simulink model "xue_flatness"  (R2017b)
settings: Solver=VariableStepAuto  StartTime=0.0  StopTime=58  RelTol=1e-9
libraries: simulink x1
(part 2 of 3)

== matlab function xue_flatness/References ==
  data: t input; references output size=18
function references = fcn(t)
%% specify your references here
g=9.81;
if t>=0 && t<2
tanalpha=-1;
if t>=0 && t<1
   [ax_d, az_d, ax_d_dot, az_d_dot, ax_d_dot_dot, az_d_dot_dot]=nest(t);
    ax_d=2/3*ax_d;                   az_d=2/3*az_d;
    ax_d_dot=2/3*ax_d_dot;           az_d_dot=2/3*az_d_dot;
    ax_d_dot_dot=2/3*ax_d_dot_dot;   az_d_dot_dot=2/3*az_d_dot_dot;
else % t>=1 && t<2
   [ax_d, az_d, ax_d_dot, az_d_dot, ax_d_dot_dot, az_d_dot_dot]=nest(t-1);
  ax_d=-2/3*ax_d;                 az_d=-2/3*az_d; % invert the direction for the sake of making end velocity zero
  ax_d_dot=-2/3*ax_d_dot;         az_d_dot=-2/3*az_d_dot;
  ax_d_dot_dot=-2/3*ax_d_dot_dot; az_d_dot_dot=-2/3*az_d_dot_dot;   
end  
 r_desired=[0 0 0]'    ;              % reference's positions is not solved here
 r_desired_dot=[0 0 0]'    ;          % reference's velocities is not solved here
 r_desired_dot_dot=[ax_d 0 az_d]'   ;       % reference's accelerations
 r_desired_dot_dot_dot=[ax_d_dot 0 az_d_dot]';      % jerk
 r_desired_dot_dot_dot_dot=[ax_d_dot_dot 0 az_d_dot_dot]' ; % snap
 psi_desired=0 ;                      % reference's yaw angle
 psi_desired_dot=0 ;                  % reference's change rate of yaw angle       
 psi_desired_dot_dot=0;
 
elseif t>=2 && t<4
r_desired=[0 0 0]'    ;              % reference's positions is not solved here
r_desired_dot=[0 0 0]'    ;          % reference's velocities is not solved here
r_desired_dot_dot=[0 0 0]'   ;       % reference's accelerations
r_desired_dot_dot_dot=[0 0 0]';      % jerk
r_desired_dot_dot_dot_dot=[0 0 0]' ; % snap
if t>=2 && t<3
psi_desired=pi/4*(t-2)^2 ;                      % reference's yaw angle
psi_desired_dot=pi/2*(t-2);                  % reference's change rate of yaw angle       
psi_desired_dot_dot=pi/2; 
else % t>=3 && t<4
psi_desired=-pi/4*(t-4)^2+pi/2 ;                      % reference's yaw angle
psi_desired_dot=-pi/2*(t-4);                  % reference's change rate of yaw angle       
psi_desired_dot_dot=-pi/2; 
end

elseif t>=4 && t<6
tanalpha=1;
if t>=4 && t<5
   [ax_d, az_d, ax_d_dot, az_d_dot, ax_d_dot_dot, az_d_dot_dot]=nest(t-4);
    ax_d=2/3*ax_d;                   az_d=2/3*az_d;
    ax_d_dot=2/3*ax_d_dot;           az_d_dot=2/3*az_d_dot;
    ax_d_dot_dot=2/3*ax_d_dot_dot;   az_d_dot_dot=2/3*az_d_dot_dot;
else % t>=5 && t<6
   [ax_d, az_d, ax_d_dot, az_d_dot, ax_d_dot_dot, az_d_dot_dot]=nest(t-5);
  ax_d=-2/3*ax_d;                 az_d=-2/3*az_d; % invert the direction for the sake of making end velocity zero
  ax_d_dot=-2/3*ax_d_dot;         az_d_dot=-2/3*az_d_dot;
  ax_d_dot_dot=-2/3*ax_d_dot_dot; az_d_dot_dot=-2/3*az_d_dot_dot;   
end  
 r_desired=[0 0 0]'    ;              % reference's positions is not solved here
 r_desired_dot=[0 0 0]'    ;          % reference's velocities is not solved here
 r_desired_dot_dot=[ax_d 0 az_d]'   ;       % reference's accelerations
 r_desired_dot_dot_dot=[ax_d_dot 0 az_d_dot]';      % jerk
 r_desired_dot_dot_dot_dot=[ax_d_dot_dot 0 az_d_dot_dot]' ; % snap
 psi_desired=pi/2 ;                      % reference's yaw angle
 psi_desired_dot=0 ;                  % reference's change rate of yaw angle       
 psi_desired_dot_dot=0;

elseif t>=6 && t<8
r_desired=[0 0 0]'    ;              % reference's positions is not solved here
r_desired_dot=[0 0 0]'    ;          % reference's velocities is not solved here
r_desired_dot_dot=[0 0 0]'   ;       % reference's accelerations
r_desired_dot_dot_dot=[0 0 0]';      % jerk
r_desired_dot_dot_dot_dot=[0 0 0]' ; % snap
if t>=6 && t<7
psi_desired=pi/2-pi/4*(t-6)^2 ;                      % reference's yaw angle
psi_desired_dot=-pi/2*(t-6);                  % reference's change rate of yaw angle       
psi_desired_dot_dot=-pi/2; 
else % t>=7 & t<8
psi_desired=pi/4*(t-8)^2 ;                      % reference's yaw angle
psi_desired_dot=pi/2*(t-8);                  % reference's change rate of yaw angle       
psi_desired_dot_dot=pi/2; 
end

elseif t>=8 && t<10
tanalpha=-1;
if t>=8 && t<9
   [ax_d, az_d, ax_d_dot, az_d_dot, ax_d_dot_dot, az_d_dot_dot]=nest(t-8);
    ax_d=2/3*ax_d;                   az_d=2/3*az_d;
    ax_d_dot=2/3*ax_d_dot;           az_d_dot=2/3*az_d_dot;
    ax_d_dot_dot=2/3*ax_d_dot_dot;   az_d_dot_dot=2/3*az_d_dot_dot;
else % t>=9 && t<10
   [ax_d, az_d, ax_d_dot, az_d_dot, ax_d_dot_dot, az_d_dot_dot]=nest(t-9);
  ax_d=-2/3*ax_d;                 az_d=-2/3*az_d; % invert the direction for the sake of making end velocity zero
  ax_d_dot=-2/3*ax_d_dot;         az_d_dot=-2/3*az_d_dot;
  ax_d_dot_dot=-2/3*ax_d_dot_dot; az_d_dot_dot=-2/3*az_d_dot_dot;   
end  
 r_desired=[0 0 0]'    ;              % reference's positions is not solved here
 r_desired_dot=[0 0 0]'    ;          % reference's velocities is not solved here
 r_desired_dot_dot=[ax_d 0 az_d]'   ;       % reference's accelerations
 r_desired_dot_dot_dot=[ax_d_dot 0 az_d_dot]';      % jerk
 r_desired_dot_dot_dot_dot=[ax_d_dot_dot 0 az_d_dot_dot]' ; % snap
 psi_desired=0 ;                      % reference's yaw angle
 psi_desired_dot=0 ;                  % reference's change rate of yaw angle       
 psi_desired_dot_dot=0;
 
elseif t>=10 && t<12
r_desired=[0 0 0]'    ;              % reference's positions is not solved here
r_desired_dot=[0 0 0]'    ;          % reference's velocities is not solved here
r_desired_dot_dot=[0 0 0]'   ;       % reference's accelerations
r_desired_dot_dot_dot=[0 0 0]';      % jerk
r_desired_dot_dot_dot_dot=[0 0 0]' ; % snap
if t>=10 && t<11
psi_desired=pi/4*(t-10)^2 ;                      % reference's yaw angle
psi_desired_dot=pi/2*(t-10);                  % reference's change rate of yaw angle       
psi_desired_dot_dot=pi/2; 
else % t>=11 && t<12
psi_desired=-pi/4*(t-12)^2+pi/2 ;                      % reference's yaw angle
psi_desired_dot=-pi/2*(t-12);                  % reference's change rate of yaw angle       
psi_desired_dot_dot=-pi/2; 
end

elseif t>=12 && t<14
tanalpha=0.5;
if t>=12 && t<13
   [ax_d, az_d, ax_d_dot, az_d_dot, ax_d_dot_dot, az_d_dot_dot]=nest(t-12);
    ax_d=406/329*ax_d;                   az_d=406/329*az_d;
    ax_d_dot=406/329*ax_d_dot;           az_d_dot=406/329*az_d_dot;
    ax_d_dot_dot=406/329*ax_d_dot_dot;   az_d_dot_dot=406/329*az_d_dot_dot;
else % t>=13 && t<14
   [ax_d, az_d, ax_d_dot, az_d_dot, ax_d_dot_dot, az_d_dot_dot]=nest(t-13);
  ax_d=-406/329*ax_d;                 az_d=-406/329*az_d; % invert the direction for the sake of making end velocity zero
  ax_d_dot=-406/329*ax_d_dot;         az_d_dot=-406/329*az_d_dot;
  ax_d_dot_dot=-406/329*ax_d_dot_dot; az_d_dot_dot=-406/329*az_d_dot_dot;   
end  
 r_desired=[0 0 0]'    ;              % reference's positions is not solved here
 r_desired_dot=[0 0 0]'    ;          % reference's velocities is not solved here
 r_desired_dot_dot=[ax_d 0 az_d]'   ;       % reference's accelerations
 r_desired_dot_dot_dot=[ax_d_dot 0 az_d_dot]';      % jerk
 r_desired_dot_dot_dot_dot=[ax_d_dot_dot 0 az_d_dot_dot]' ; % snap
 psi_desired=pi/2 ;                      % reference's yaw angle
 psi_desired_dot=0 ;                  % reference's change rate of yaw angle       
 psi_desired_dot_dot=0;
 
elseif t>=14 && t<16
r_desired=[0 0 0]'    ;              % reference's positions is not solved here
r_desired_dot=[0 0 0]'    ;          % reference's velocities is not solved here
r_desired_dot_dot=[0 0 0]'   ;       % reference's accelerations
r_desired_dot_dot_dot=[0 0 0]';      % jerk
r_desired_dot_dot_dot_dot=[0 0 0]' ; % snap
if t>=14 && t<15
psi_desired=pi/2-pi/4*(t-14)^2 ;                      % reference's yaw angle
psi_desired_dot=-pi/2*(t-14);                  % reference's change rate of yaw angle       
psi_desired_dot_dot=-pi/2; 
else % t>=15 & t<16
psi_desired=pi/4*(t-16)^2 ;                      % reference's yaw angle
psi_desired_dot=pi/2*(t-16);                  % reference's change rate of yaw angle       
psi_desired_dot_dot=pi/2; 
end    

elseif t>=16 && t<18
tanalpha=1;
if t>=16 && t<17
   [ax_d, az_d, ax_d_dot, az_d_dot, ax_d_dot_dot, az_d_dot_dot]=nest(t-16);
    ax_d=-2/3*ax_d;                   az_d=-2/3*az_d;
    ax_d_dot=-2/3*ax_d_dot;           az_d_dot=-2/3*az_d_dot;
    ax_d_dot_dot=-2/3*ax_d_dot_dot;   az_d_dot_dot=-2/3*az_d_dot_dot;
else % t>=17 && t<18
   [ax_d, az_d, ax_d_dot, az_d_dot, ax_d_dot_dot, az_d_dot_dot]=nest(t-17);
  ax_d=2/3*ax_d;                 az_d=2/3*az_d; % invert the direction for the sake of making end velocity zero
  ax_d_dot=2/3*ax_d_dot;         az_d_dot=2/3*az_d_dot;
  ax_d_dot_dot=2/3*ax_d_dot_dot; az_d_dot_dot=2/3*az_d_dot_dot;   
end  
 r_desired=[0 0 0]'    ;              % reference's positions is not solved here
 r_desired_dot=[0 0 0]'    ;          % reference's velocities is not solved here
 r_desired_dot_dot=[ax_d 0 az_d]'   ;       % reference's accelerations
 r_desired_dot_dot_dot=[ax_d_dot 0 az_d_dot]';      % jerk
 r_desired_dot_dot_dot_dot=[ax_d_dot_dot 0 az_d_dot_dot]' ; % snap
 psi_desired=0 ;                      % reference's yaw angle
 psi_desired_dot=0 ;                  % reference's change rate of yaw angle       
 psi_desired_dot_dot=0;   
 
elseif t>=18 && t<20
r_desired=[0 0 0]'    ;              % reference's positions is not solved here
r_desired_dot=[0 0 0]'    ;          % reference's velocities is not solved here
r_desired_dot_dot=[0 0 0]'   ;       % reference's accelerations
r_desired_dot_dot_dot=[0 0 0]';      % jerk
r_desired_dot_dot_dot_dot=[0 0 0]' ; % snap
if t>=18 && t<19
psi_desired=pi/4*(t-18)^2 ;                      % reference's yaw angle
psi_desired_dot=pi/2*(t-18);                  % reference's change rate of yaw angle       
psi_desired_dot_dot=pi/2; 
else % t>=19 && t<20
psi_desired=-pi/4*(t-20)^2+pi/2 ;                      % reference's yaw angle
psi_desired_dot=-pi/2*(t-20);                  % reference's change rate of yaw angle       
psi_desired_dot_dot=-pi/2; 
end

elseif t>=20 && t<22
tanalpha=1/8;
if t>=20 && t<21
   [ax_d, az_d, ax_d_dot, az_d_dot, ax_d_dot_dot, az_d_dot_dot]=nest(t-20);
    ax_d=-8/3*ax_d;                   az_d=-8/3*az_d;
    ax_d_dot=-8/3*ax_d_dot;           az_d_dot=-8/3*az_d_dot;
    ax_d_dot_dot=-8/3*ax_d_dot_dot;   az_d_dot_dot=-8/3*az_d_dot_dot;
else % t>=21 && t<22
   [ax_d, az_d, ax_d_dot, az_d_dot, ax_d_dot_dot, az_d_dot_dot]=nest(t-21);
  ax_d=8/3*ax_d;                 az_d=8/3*az_d; % invert the direction for the sake of making end velocity zero
  ax_d_dot=8/3*ax_d_dot;         az_d_dot=8/3*az_d_dot;
  ax_d_dot_dot=8/3*ax_d_dot_dot; az_d_dot_dot=8/3*az_d_dot_dot;   
end  
 r_desired=[0 0 0]'    ;              % reference's positions is not solved here
 r_desired_dot=[0 0 0]'    ;          % reference's velocities is not solved here
 r_desired_dot_dot=[ax_d 0 az_d]'   ;       % reference's accelerations
 r_desired_dot_dot_dot=[ax_d_dot 0 az_d_dot]';      % jerk
 r_desired_dot_dot_dot_dot=[ax_d_dot_dot 0 az_d_dot_dot]' ; % snap
 psi_desired=pi/2 ;                      % reference's yaw angle
 psi_desired_dot=0 ;                  % reference's change rate of yaw angle       
 psi_desired_dot_dot=0; 
 
elseif t>=22 && t<24
r_desired=[0 0 0]'    ;              % reference's positions is not solved here
r_desired_dot=[0 0 0]'    ;          % reference's velocities is not solved here
r_desired_dot_dot=[0 0 0]'   ;       % reference's accelerations
r_desired_dot_dot_dot=[0 0 0]';      % jerk
r_desired_dot_dot_dot_dot=[0 0 0]' ; % snap
if t>=22 && t<23
psi_desired=pi/2-pi/4*(t-22)^2 ;                      % reference's yaw angle
psi_desired_dot=-pi/2*(t-22);                  % reference's change rate of yaw angle       
psi_desired_dot_dot=-pi/2; 
else % t>=23 & t<24
psi_desired=pi/4*(t-24)^2 ;                      % reference's yaw angle
psi_desired_dot=pi/2*(t-24);                  % reference's change rate of yaw angle       
psi_desired_dot_dot=pi/2; 
end

elseif t>=24 && t<26
if t>=24 && t<25
 r_desired=[0 0 0]'    ;              % reference's positions 
 r_desired_dot=[0 0 0]'    ;          % reference's velocities
 r_desired_dot_dot=[0 0 -1/4]'   ;       % reference's accelerations
 r_desired_dot_dot_dot=[0 0 0]';      % jerk
 r_desired_dot_dot_dot_dot=[0 0 0]' ; % snap
else
 r_desired=[0 0 0]'    ;     % reference's positions 
 r_desired_dot=[0 0 0]'    ;   % reference's velocities 
 r_desired_dot_dot=[0 0 1/4]'   ;       % reference's accelerations
 r_desired_dot_dot_dot=[0 0 0]';      % jerk
 r_desired_dot_dot_dot_dot=[0 0 0]' ; % snap
end
 psi_desired=0 ;                      % reference's yaw angle
 psi_desired_dot=0 ;                  % reference's change rate of yaw angle       
 psi_desired_dot_dot=0;
 
elseif t>=26 && t<28
r_desired=[0 0 0]'    ;              % reference's positions is not solved here
r_desired_dot=[0 0 0]'    ;          % reference's velocities is not solved here
r_desired_dot_dot=[0 0 0]'   ;       % reference's accelerations
r_desired_dot_dot_dot=[0 0 0]';      % jerk
r_desired_dot_dot_dot_dot=[0 0 0]' ; % snap
if t>=26 && t<27
psi_desired=pi/4*(t-26)^2 ;                      % reference's yaw angle
psi_desired_dot=pi/2*(t-26);                  % reference's change rate of yaw angle       
psi_desired_dot_dot=pi/2; 
else % t>=27 && t<28
psi_desired=-pi/4*(t-28)^2+pi/2 ;                      % reference's yaw angle
psi_desired_dot=-pi/2*(t-28);                  % reference's change rate of yaw angle       
psi_desired_dot_dot=-pi/2; 
end

elseif t>=28 && t<30
if t>=28 && t<29
 r_desired=[0 0 0]'    ;              % reference's positions 
 r_desired_dot=[0 0 0]'    ;          % reference's velocities
 r_desired_dot_dot=[0 0 1/4]'   ;       % reference's accelerations
 r_desired_dot_dot_dot=[0 0 0]';      % jerk
 r_desired_dot_dot_dot_dot=[0 0 0]' ; % snap
else
 r_desired=[0 0 0]'    ;     % reference's positions 
 r_desired_dot=[0 0 0]'    ;   % reference's velocities 
 r_desired_dot_dot=[0 0 -1/4]'   ;       % reference's accelerations
 r_desired_dot_dot_dot=[0 0 0]';      % jerk
 r_desired_dot_dot_dot_dot=[0 0 0]' ; % snap
end
 psi_desired=pi/2 ;                      % reference's yaw angle
 psi_desired_dot=0 ;                  % reference's change rate of yaw angle       
 psi_desired_dot_dot=0;
 
elseif t>=30 && t<32
r_desired=[0 0 0]'    ;              % reference's positions is not solved here
r_desired_dot=[0 0 0]'    ;          % reference's velocities is not solved here
r_desired_dot_dot=[0 0 0]'   ;       % reference's accelerations
r_desired_dot_dot_dot=[0 0 0]';      % jerk
r_desired_dot_dot_dot_dot=[0 0 0]' ; % snap
if t>=30 && t<31
psi_desired=pi/2-pi/4*(t-30)^2 ;                      % reference's yaw angle
psi_desired_dot=-pi/2*(t-30);                  % reference's change rate of yaw angle       
psi_desired_dot_dot=-pi/2; 
else % t>=31 & t<32
psi_desired=pi/4*(t-32)^2 ;                      % reference's yaw angle
psi_desired_dot=pi/2*(t-32);                  % reference's change rate of yaw angle       
psi_desired_dot_dot=pi/2; 
end

elseif t>=32 && t<34
tanalpha=0;
if t>=32 && t<33
   [ax_d, az_d, ax_d_dot, az_d_dot, ax_d_dot_dot, az_d_dot_dot]=nest(t-32);
    ax_d=3.5*ax_d;                   az_d=3.5*az_d;
    ax_d_dot=3.5*ax_d_dot;           az_d_dot=3.5*az_d_dot;
    ax_d_dot_dot=3.5*ax_d_dot_dot;   az_d_dot_dot=3.5*az_d_dot_dot;
else % t>=33 && t<34
   [ax_d, az_d, ax_d_dot, az_d_dot, ax_d_dot_dot, az_d_dot_dot]=nest(t-33);
  ax_d=-3.5*ax_d;                 az_d=-3.5*az_d; % invert the direction for the sake of making end velocity zero
  ax_d_dot=-3.5*ax_d_dot;         az_d_dot=-3.5*az_d_dot;
  ax_d_dot_dot=-3.5*ax_d_dot_dot; az_d_dot_dot=-3.5*az_d_dot_dot;   
end  
 r_desired=[0 0 0]'    ;              % reference's positions is not solved here
 r_desired_dot=[0 0 0]'    ;          % reference's velocities is not solved here
 r_desired_dot_dot=[ax_d 0 az_d]'   ;       % reference's accelerations
 r_desired_dot_dot_dot=[ax_d_dot 0 az_d_dot]';      % jerk
 r_desired_dot_dot_dot_dot=[ax_d_dot_dot 0 az_d_dot_dot]' ; % snap
 psi_desired=0 ;                      % reference's yaw angle
 psi_desired_dot=0 ;                  % reference's change rate of yaw angle       
 psi_desired_dot_dot=0;
 
elseif t>=34 && t<36
if t>=34 && t<35
 r_desired=[0 0 0]'    ;              % reference's positions 
 r_desired_dot=[0 0 0]'    ;          % reference's velocities
 r_desired_dot_dot=[0 0 -1/4]'   ;       % reference's accelerations
 r_desired_dot_dot_dot=[0 0 0]';      % jerk
 r_desired_dot_dot_dot_dot=[0 0 0]' ; % snap
else
 r_desired=[0 0 0]'    ;     % reference's positions 
 r_desired_dot=[0 0 0]'    ;   % reference's velocities 
 r_desired_dot_dot=[0 0 1/4]'   ;       % reference's accelerations
 r_desired_dot_dot_dot=[0 0 0]';      % jerk
 r_desired_dot_dot_dot_dot=[0 0 0]' ; % snap
end
 psi_desired=0 ;                      % reference's yaw angle
 psi_desired_dot=0 ;                  % reference's change rate of yaw angle       
 psi_desired_dot_dot=0;
 
elseif t>=36 && t<38
r_desired=[0 0 0]'    ;              % reference's positions is not solved here
r_desired_dot=[0 0 0]'    ;          % reference's velocities is not solved here
r_desired_dot_dot=[0 0 0]'   ;       % reference's accelerations
r_desired_dot_dot_dot=[0 0 0]';      % jerk
r_desired_dot_dot_dot_dot=[0 0 0]' ; % snap
if t>=36 && t<37
psi_desired=pi/4*(t-36)^2 ;                      % reference's yaw angle
psi_desired_dot=pi/2*(t-36);                  % reference's change rate of yaw angle       
psi_desired_dot_dot=pi/2; 
else % t>=37 && t<38
psi_desired=-pi/4*(t-38)^2+pi/2 ;                      % reference's yaw angle
psi_desired_dot=-pi/2*(t-38);                  % reference's change rate of yaw angle       
psi_desired_dot_dot=-pi/2; 
end

elseif t>=38 && t<40
tanalpha=0;
if t>=38 && t<39
   [ax_d, az_d, ax_d_dot, az_d_dot, ax_d_dot_dot, az_d_dot_dot]=nest(t-38);
    ax_d=-3*ax_d;                   az_d=-3*az_d;
    ax_d_dot=-3*ax_d_dot;           az_d_dot=-3*az_d_dot;
    ax_d_dot_dot=-3*ax_d_dot_dot;   az_d_dot_dot=-3*az_d_dot_dot;
else % t>=39 && t<40
   [ax_d, az_d, ax_d_dot, az_d_dot, ax_d_dot_dot, az_d_dot_dot]=nest(t-39);
  ax_d=3*ax_d;                 az_d=3*az_d; % invert the direction for the sake of making end velocity zero
  ax_d_dot=3*ax_d_dot;         az_d_dot=3*az_d_dot;
  ax_d_dot_dot=3*ax_d_dot_dot; az_d_dot_dot=3*az_d_dot_dot;   
end  
 r_desired=[0 0 0]'    ;              % reference's positions is not solved here
 r_desired_dot=[0 0 0]'    ;          % reference's velocities is not solved here
 r_desired_dot_dot=[ax_d 0 az_d]'   ;       % reference's accelerations
 r_desired_dot_dot_dot=[ax_d_dot 0 az_d_dot]';      % jerk
 r_desired_dot_dot_dot_dot=[ax_d_dot_dot 0 az_d_dot_dot]' ; % snap
 psi_desired=pi/2 ;                      % reference's yaw angle
 psi_desired_dot=0 ;                  % reference's change rate of yaw angle       
 psi_desired_dot_dot=0;
 
elseif t>=40 && t<42
r_desired=[0 0 0]'    ;              % reference's positions is not solved here
r_desired_dot=[0 0 0]'    ;          % reference's velocities is not solved here
r_desired_dot_dot=[0 0 0]'   ;       % reference's accelerations
r_desired_dot_dot_dot=[0 0 0]';      % jerk
r_desired_dot_dot_dot_dot=[0 0 0]' ; % snap
if t>=40 && t<41
psi_desired=pi/2-pi/4*(t-40)^2 ;                      % reference's yaw angle
psi_desired_dot=-pi/2*(t-40);                  % reference's change rate of yaw angle       
psi_desired_dot_dot=-pi/2; 
else % t>=41 & t<42
psi_desired=pi/4*(t-42)^2 ;                      % reference's yaw angle
psi_desired_dot=pi/2*(t-42);                  % reference's change rate of yaw angle       
psi_desired_dot_dot=pi/2; 
end 

elseif t>=42 && t<44
tanalpha=0;
if t>=42 && t<43
   [ax_d, az_d, ax_d_dot, az_d_dot, ax_d_dot_dot, az_d_dot_dot]=nest(t-42);
    ax_d=2.5*ax_d;                   az_d=2.5*az_d;
    ax_d_dot=2.5*ax_d_dot;           az_d_dot=2.5*az_d_dot;
    ax_d_dot_dot=2.5*ax_d_dot_dot;   az_d_dot_dot=2.5*az_d_dot_dot;
else % t>=43 && t<44
   [ax_d, az_d, ax_d_dot, az_d_dot, ax_d_dot_dot, az_d_dot_dot]=nest(t-43);
  ax_d=-2.5*ax_d;                 az_d=-2.5*az_d; % invert the direction for the sake of making end velocity zero
  ax_d_dot=-2.5*ax_d_dot;         az_d_dot=-2.5*az_d_dot;
  ax_d_dot_dot=-2.5*ax_d_dot_dot; az_d_dot_dot=-2.5*az_d_dot_dot;   
end  
 r_desired=[0 0 0]'    ;              % reference's positions is not solved here
 r_desired_dot=[0 0 0]'    ;          % reference's velocities is not solved here
 r_desired_dot_dot=[ax_d 0 az_d]'   ;       % reference's accelerations
 r_desired_dot_dot_dot=[ax_d_dot 0 az_d_dot]';      % jerk
 r_desired_dot_dot_dot_dot=[ax_d_dot_dot 0 az_d_dot_dot]' ; % snap
 psi_desired=0 ;                      % reference's yaw angle
 psi_desired_dot=0 ;                  % reference's change rate of yaw angle       
 psi_desired_dot_dot=0;  
 
elseif t>=44 && t<46
tanalpha=1/2;
if t>=44 && t<45
   [ax_d, az_d, ax_d_dot, az_d_dot, ax_d_dot_dot, az_d_dot_dot]=nest(t-44);
    ax_d=-5/4*ax_d;                   az_d=-5/4*az_d;
    ax_d_dot=-5/4*ax_d_dot;           az_d_dot=-5/4*az_d_dot;
    ax_d_dot_dot=-5/4*ax_d_dot_dot;   az_d_dot_dot=-5/4*az_d_dot_dot;
else % t>=45 && t<46
   [ax_d, az_d, ax_d_dot, az_d_dot, ax_d_dot_dot, az_d_dot_dot]=nest(t-45);
  ax_d=5/4*ax_d;                 az_d=5/4*az_d; % invert the direction for the sake of making end velocity zero
  ax_d_dot=5/4*ax_d_dot;         az_d_dot=5/4*az_d_dot;
  ax_d_dot_dot=5/4*ax_d_dot_dot; az_d_dot_dot=5/4*az_d_dot_dot;   
end  
 r_desired=[0 0 0]'    ;              % reference's positions is not solved here
 r_desired_dot=[0 0 0]'    ;          % reference's velocities is not solved here
 r_desired_dot_dot=[ax_d 0 az_d]'   ;       % reference's accelerations
 r_desired_dot_dot_dot=[ax_d_dot 0 az_d_dot]';      % jerk
 r_desired_dot_dot_dot_dot=[ax_d_dot_dot 0 az_d_dot_dot]' ; % snap
 psi_desired=0 ;                      % reference's yaw angle
 psi_desired_dot=0 ;                  % reference's change rate of yaw angle       
 psi_desired_dot_dot=0;  
 
elseif t>=46 && t<48
if t>=46 && t<47
 r_desired=[0 0 0]'    ;              % reference's positions 
 r_desired_dot=[0 0 0]'    ;          % reference's velocities
 r_desired_dot_dot=[0 0 -1/2]'   ;       % reference's accelerations
 r_desired_dot_dot_dot=[0 0 0]';      % jerk
 r_desired_dot_dot_dot_dot=[0 0 0]' ; % snap
else
 r_desired=[0 0 0]'    ;     % reference's positions 
 r_desired_dot=[0 0 0]'    ;   % reference's velocities 
 r_desired_dot_dot=[0 0 1/2]'   ;       % reference's accelerations
 r_desired_dot_dot_dot=[0 0 0]';      % jerk
 r_desired_dot_dot_dot_dot=[0 0 0]' ; % snap
end
 psi_desired=0 ;                      % reference's yaw angle
 psi_desired_dot=0 ;                  % reference's change rate of yaw angle       
 psi_desired_dot_dot=0;
 
elseif t>=48 && t<50
tanalpha=-1/2;
if t>=48 && t<49
   [ax_d, az_d, ax_d_dot, az_d_dot, ax_d_dot_dot, az_d_dot_dot]=nest(t-48);
    ax_d=-ax_d;                   az_d=-az_d;
    ax_d_dot=-ax_d_dot;           az_d_dot=-az_d_dot;
    ax_d_dot_dot=-ax_d_dot_dot;   az_d_dot_dot=-az_d_dot_dot;
else % t>=49 && t<50
   [ax_d, az_d, ax_d_dot, az_d_dot, ax_d_dot_dot, az_d_dot_dot]=nest(t-49);
  ax_d=ax_d;                 az_d=az_d; % invert the direction for the sake of making end velocity zero
  ax_d_dot=ax_d_dot;         az_d_dot=az_d_dot;
  ax_d_dot_dot=ax_d_dot_dot; az_d_dot_dot=az_d_dot_dot;   
end  
 r_desired=[0 0 0]'    ;              % reference's positions is not solved here
 r_desired_dot=[0 0 0]'    ;          % reference's velocities is not solved here
 r_desired_dot_dot=[ax_d 0 az_d]'   ;       % reference's accelerations
 r_desired_dot_dot_dot=[ax_d_dot 0 az_d_dot]';      % jerk
 r_desired_dot_dot_dot_dot=[ax_d_dot_dot 0 az_d_dot_dot]' ; % snap
 psi_desired=0 ;                      % reference's yaw angle
 psi_desired_dot=0 ;                  % reference's change rate of yaw angle       
 psi_desired_dot_dot=0;   
 
elseif t>=50 && t<52
r_desired=[0 0 0]'    ;              % reference's positions is not solved here
r_desired_dot=[0 0 0]'    ;          % reference's velocities is not solved here
r_desired_dot_dot=[0 0 0]'   ;       % reference's accelerations
r_desired_dot_dot_dot=[0 0 0]';      % jerk
r_desired_dot_dot_dot_dot=[0 0 0]' ; % snap
if t>=50 && t<51
psi_desired=pi/4*(t-50)^2 ;                      % reference's yaw angle
psi_desired_dot=pi/2*(t-50);                  % reference's change rate of yaw angle       
psi_desired_dot_dot=pi/2; 
else % t>=51 && t<52
psi_desired=-pi/4*(t-52)^2+pi/2 ;                      % reference's yaw angle
psi_desired_dot=-pi/2*(t-52);                  % reference's change rate of yaw angle       
psi_desired_dot_dot=-pi/2; 
end

elseif t>=52 && t<54
tanalpha=-1;
if t>=52 && t<53
   [ax_d, az_d, ax_d_dot, az_d_dot, ax_d_dot_dot, az_d_dot_dot]=nest(t-52);
    ax_d=-ax_d;                   az_d=-az_d;
    ax_d_dot=-ax_d_dot;           az_d_dot=-az_d_dot;
    ax_d_dot_dot=-ax_d_dot_dot;   az_d_dot_dot=-az_d_dot_dot;
else % t>=53 && t<54
   [ax_d, az_d, ax_d_dot, az_d_dot, ax_d_dot_dot, az_d_dot_dot]=nest(t-53);
  ax_d=ax_d;                 az_d=az_d; % invert the direction for the sake of making end velocity zero
  ax_d_dot=ax_d_dot;         az_d_dot=az_d_dot;
  ax_d_dot_dot=ax_d_dot_dot; az_d_dot_dot=az_d_dot_dot;   
end  
 r_desired=[0 0 0]'    ;              % reference's positions is not solved here
 r_desired_dot=[0 0 0]'    ;          % reference's velocities is not solved here
 r_desired_dot_dot=[ax_d 0 az_d]'   ;       % reference's accelerations
 r_desired_dot_dot_dot=[ax_d_dot 0 az_d_dot]';      % jerk
 r_desired_dot_dot_dot_dot=[ax_d_dot_dot 0 az_d_dot_dot]' ; % snap
 psi_desired=pi/2 ;                      % reference's yaw angle
 psi_desired_dot=0 ;                  % reference's change rate of yaw angle       
 psi_desired_dot_dot=0;  
 
elseif t>=54 && t<56
r_desired=[0 0 0]'    ;              % reference's positions is not solved here
r_desired_dot=[0 0 0]'    ;          % reference's velocities is not solved here
r_desired_dot_dot=[0 0 0]'   ;       % reference's accelerations
r_desired_dot_dot_dot=[0 0 0]';      % jerk
r_desired_dot_dot_dot_dot=[0 0 0]' ; % snap
if t>=54 && t<55
psi_desired=pi/2-pi/4*(t-54)^2 ;                      % reference's yaw angle
psi_desired_dot=-pi/2*(t-54);                  % reference's change rate of yaw angle       
psi_desired_dot_dot=-pi/2; 
else % t>=55 & t<56
psi_desired=pi/4*(t-56)^2 ;                      % reference's yaw angle
psi_desired_dot=pi/2*(t-56);                  % reference's change rate of yaw angle       
psi_desired_dot_dot=pi/2; 
end

else
tanalpha=0;
if t>=56 && t<57
   [ax_d, az_d, ax_d_dot, az_d_dot, ax_d_dot_dot, az_d_dot_dot]=nest(t-56);
    ax_d=4*ax_d;                   az_d=4*az_d;
    ax_d_dot=4*ax_d_dot;           az_d_dot=4*az_d_dot;
    ax_d_dot_dot=4*ax_d_dot_dot;   az_d_dot_dot=4*az_d_dot_dot;
else % t>=57 && t<58
   [ax_d, az_d, ax_d_dot, az_d_dot, ax_d_dot_dot, az_d_dot_dot]=nest(t-57);
  ax_d=-4*ax_d;                 az_d=-4*az_d; % invert the direction for the sake of making end velocity zero
  ax_d_dot=-4*ax_d_dot;         az_d_dot=-4*az_d_dot;
  ax_d_dot_dot=-4*ax_d_dot_dot; az_d_dot_dot=-4*az_d_dot_dot;   
end  
 r_desired=[0 0 0]'    ;              % reference's positions is not solved here
 r_desired_dot=[0 0 0]'    ;          % reference's velocities is not solved here
 r_desired_dot_dot=[ax_d 0 az_d]'   ;       % reference's accelerations
 r_desired_dot_dot_dot=[ax_d_dot 0 az_d_dot]';      % jerk
 r_desired_dot_dot_dot_dot=[ax_d_dot_dot 0 az_d_dot_dot]' ; % snap
 psi_desired=0 ;                      % reference's yaw angle
 psi_desired_dot=0 ;                  % reference's change rate of yaw angle       
 psi_desired_dot_dot=0; 
end
 
  function   [axn, azn, axn_dot, azn_dot, axn_dot_dot, azn_dot_dot]=nest(tn)
        if tn>=0 && tn<1/4
        angle=pi/6*tn^2;               angle_dot=pi/3*tn;           angle_dot_dot=pi/3;
        elseif tn>=1/4 && tn<3/4
        angle=-pi/6*(tn-1/2)^2+pi/48;  angle_dot=-pi/3*(tn-1/2);    angle_dot_dot=-pi/3;
        else 
        angle=pi/6*(tn-1)^2;           angle_dot=pi/3*(tn-1);       angle_dot_dot=pi/3;
        end
     axn=g*tan(angle)/(1-tanalpha*tan(angle));
     azn=tanalpha*axn;
     axn_dot=g*(1+tan(angle)^2)*angle_dot/(1-tanalpha*tan(angle))^2;
     azn_dot=tanalpha*axn_dot;
     axn_dot_dot=g*(1+tan(angle)^2)*(2*angle_dot^2*(tan(angle)+tanalpha)+angle_dot_dot*(1-tanalpha*tan(angle)))/(1-tanalpha*tan(angle))^3;
     azn_dot_dot=tanalpha*axn_dot_dot;
  end
references=[r_desired;                 %  1-3
            r_desired_dot;             %  4-6
            r_desired_dot_dot;         %  7-9
            r_desired_dot_dot_dot;     %  10-12
            r_desired_dot_dot_dot_dot; %  13-15
            psi_desired;               %  16
            psi_desired_dot;           %  17
            psi_desired_dot_dot];      %  18
end
%% sources
%% -------- a horizontal circle with radius of 3 m-------------------------------
% r_desired=[3*cos(t) 3*sin(t) 0]'    ;             % reference's positions
% r_desired_dot=[-3*sin(t) 3*cos(t) 0]'    ;        % reference's velocities
% r_desired_dot_dot=[-3*cos(t) -3*sin(t) 0]'   ;    % reference's accelerations
% r_desired_dot_dot_dot=[3*sin(t) -3*cos(t) 0]';    % jerk
% r_desired_dot_dot_dot_dot=[3*cos(t) 3*sin(t) 0]' ;% snap
% psi_desired=0 ;                % reference's yaw angle
% psi_desired_dot=0 ;            % reference's change rate of yaw angle    
% psi_desired_dot_dot=0;
% [3 0 0,0 3 0,0 -acos(9.81/sqrt(9+9.81^2)) 0,3/sqrt(9+9.81^2) 0 0] % initial condition
%% -------- a vertiacal circle with radius of 3 m-------------------------------
% r_desired=[0 3*sin(t) -3*cos(t)]'    ;             % reference's positions
% r_desired_dot=[0 3*cos(t) 3*sin(t)]'    ;        % reference's velocities
% r_desired_dot_dot=[0 -3*sin(t) 3*cos(t)]'   ;    % reference's accelerations
% r_desired_dot_dot_dot=[0 -3*cos(t) -3*sin(t)]';    % jerk
% r_desired_dot_dot_dot_dot=[0 3*sin(t) -3*cos(t)]' ;% snap
% psi_desired=0 ;                % reference's yaw angle
% psi_desired_dot=0 ;            % reference's change rate of yaw angle    
% psi_desired_dot_dot=0;
%% ------------------a horizontal straight line--------------------------
% g=9.81;
%  if t>=0 & t<1 
%     theta_d=pi/6*t^2 ;           theta_d_dot=pi/3*t ;      theta_d_dot_dot=pi/3;
%  elseif t>=1 & t<3
%     theta_d=-pi/6*(t-2)^2+pi/3 ; theta_d_dot=-pi/3*(t-2) ; theta_d_dot_dot=-pi/3;
%  elseif t>=3 & t<4
%     theta_d=pi/6*(t-4)^2 ;       theta_d_dot=pi/3*(t-4) ;  theta_d_dot_dot=pi/3;
%  elseif t>=4 & t<5
%     theta_d=-pi/6*(t-4)^2 ;      theta_d_dot=-pi/3*(t-4) ; theta_d_dot_dot=-pi/3;
%  elseif t>=5 & t<7
%     theta_d=pi/6*(t-6)^2-pi/3 ;  theta_d_dot=pi/3*(t-6) ;  theta_d_dot_dot=pi/3;
%  else 
%     theta_d=-pi/6*(t-8)^2 ;      theta_d_dot=-pi/3*(t-8);  theta_d_dot_dot=-pi/3;
%  end
%  r_desired=[0 0 0]'    ;              % reference's positions is not solved here
%  r_desired_dot=[0 0 0]'    ;          % reference's velocities is not solved here
%  r_desired_dot_dot=[1/100*g*tan(theta_d) 0 0]'   ;       % reference's accelerations
%  r_desired_dot_dot_dot=[1/100*g*(1+tan(theta_d)^2)*theta_d_dot 0 0]';      % jerk
%  r_desired_dot_dot_dot_dot=[1/100*g*(1+tan(theta_d)^2)*(2*tan(theta_d)*theta_d_dot^2+theta_d_dot_dot) 0 0]' ; % snap
%  psi_desired=0 ;                      % reference's yaw angle
%  psi_desired_dot=0 ;                  % reference's change rate of yaw angle       
%  psi_desired_dot_dot=0;
%% ----- inclined straight line (2s)-----
% g=9.81;
% tanalpha=0 ; % slope
% if t<1
%    [ax_d az_d ax_d_dot az_d_dot ax_d_dot_dot az_d_dot_dot]=nest(t);
% else
%    [ax_d az_d ax_d_dot az_d_dot ax_d_dot_dot az_d_dot_dot]=nest(t-1);
%   ax_d=-ax_d; % invert the direction for the sake of making end velocity zero
%   az_d=-az_d;
%   ax_d_dot=-ax_d_dot;
%   az_d_dot=-az_d_dot;
%   ax_d_dot_dot=-ax_d_dot_dot;
%   az_d_dot_dot=-az_d_dot_dot;  
% end
%     function   [axn azn axn_dot azn_dot axn_dot_dot azn_dot_dot]=nest(tn)
%         if tn>=0 & tn<1/4
%         angle=8*pi/3*tn^2;               angle_dot=16*pi/3*tn;           angle_dot_dot=16*pi/3;
%         elseif tn>=1/4 & tn<3/4
%         angle=-8*pi/3*(tn-1/2)^2+pi/3;   angle_dot=-16*pi/3*(tn-1/2);    angle_dot_dot=-pi*16/3;
%         else 
%         angle=pi*8/3*(tn-1)^2;           angle_dot=pi*16/3*(tn-1);       angle_dot_dot=pi*16/3;
%         end
%      axn=g*tan(angle)/(1-tanalpha*tan(angle));
%      azn=tanalpha*axn;
%      axn_dot=g*(1+tan(angle)^2)*angle_dot/(1-tanalpha*tan(angle))^2;
%      azn_dot=tanalpha*axn_dot;
%      axn_dot_dot=g*(1+tan(angle)^2)*(2*angle_dot^2*(tan(angle)+tanalpha)+angle_dot_dot*(1-tanalpha*tan(angle)))/(1-tanalpha*tan(angle))^3;
%      azn_dot_dot=tanalpha*axn_dot_dot;
%     end
%  r_desired=[0 0 0]'    ;              % reference's positions is not solved here
%  r_desired_dot=[0 0 0]'    ;          % reference's velocities is not solved here
%  r_desired_dot_dot=[ax_d 0 az_d]'   ;       % reference's accelerations
%  r_desired_dot_dot_dot=[ax_d_dot 0 az_d_dot]';      % jerk
%  r_desired_dot_dot_dot_dot=[ax_d_dot_dot 0 az_d_dot_dot]' ; % snap
%  psi_desired=0 ;                      % reference's yaw angle
%  psi_desired_dot=0 ;                  % reference's change rate of yaw angle       
%  psi_desired_dot_dot=0;
%% ----------------inclined straight line(8s)-----------
% g=9.81;
% tanalpha=-2 ; % slope
% if t<4
%    [ax_d az_d ax_d_dot az_d_dot ax_d_dot_dot az_d_dot_dot]=nest(t);
% else
%    [ax_d az_d ax_d_dot az_d_dot ax_d_dot_dot az_d_dot_dot]=nest(t-4);
%   ax_d=-ax_d; % invert the direction for the sake of making end velocity zero
%   az_d=-az_d;
%   ax_d_dot=-ax_d_dot;
%   az_d_dot=-az_d_dot;
%   ax_d_dot_dot=-ax_d_dot_dot;
%   az_d_dot_dot=-az_d_dot_dot;  
% end
%     function   [axn azn axn_dot azn_dot axn_dot_dot azn_dot_dot]=nest(tn)
%         if tn>=0 & tn<1
%         angle=pi/6*tn^2;           angle_dot=pi/3*tn;      angle_dot_dot=pi/3;
%         elseif tn>=1 & tn<3
%         angle=-pi/6*(tn-2)^2+pi/3; angle_dot=-pi/3*(tn-2); angle_dot_dot=-pi/3;
%         else 
%         angle=pi/6*(tn-4)^2;       angle_dot=pi/3*(tn-4);  angle_dot_dot=pi/3;
%         end
%      axn=g*tan(angle)/(1-tanalpha*tan(angle));
%      azn=tanalpha*axn;
%      axn_dot=g*(1+tan(angle)^2)*angle_dot/(1-tanalpha*tan(angle))^2;
%      azn_dot=tanalpha*axn_dot;
%      axn_dot_dot=g*(1+tan(angle)^2)*(2*angle_dot^2*(tan(angle)+tanalpha)+angle_dot_dot*(1-tanalpha*tan(angle)))/(1-tanalpha*tan(angle))^3;
%      azn_dot_dot=tanalpha*axn_dot_dot;
%     end
%  r_desired=[0 0 0]'    ;              % reference's positions is not solved here
%  r_desired_dot=[0 0 0]'    ;          % reference's velocities is not solved here
%  r_desired_dot_dot=[ax_d 0 az_d]'   ;       % reference's accelerations
%  r_desired_dot_dot_dot=[ax_d_dot 0 az_d_dot]';      % jerk
%  r_desired_dot_dot_dot_dot=[ax_d_dot_dot 0 az_d_dot_dot]' ; % snap
%  psi_desired=0 ;                      % reference's yaw angle
%  psi_desired_dot=0 ;                  % reference's change rate of yaw angle       
%  psi_desired_dot_dot=0;
%% -----------a vertical straight line------------------
% if t<1
%  r_desired=[0 0 t^2]'    ;              % reference's positions 
%  r_desired_dot=[0 0 2*t]'    ;          % reference's velocities
%  r_desired_dot_dot=[0 0 2]'   ;       % reference's accelerations
%  r_desired_dot_dot_dot=[0 0 0]';      % jerk
%  r_desired_dot_dot_dot_dot=[0 0 0]' ; % snap
% else
%  r_desired=[0 0 -(t-2)^2+2]'    ;              % reference's positions 
%  r_desired_dot=[0 0 -2*(t-2)]'    ;          % reference's velocities 
%  r_desired_dot_dot=[0 0 -2]'   ;       % reference's accelerations
%  r_desired_dot_dot_dot=[0 0 0]';      % jerk
%  r_desired_dot_dot_dot_dot=[0 0 0]' ; % snap
% end
%  psi_desired=0 ;                      % reference's yaw angle
%  psi_desired_dot=0 ;                  % reference's change rate of yaw angle       
%  psi_desired_dot_dot=0;
%% --------W------------------------------------
% g=9.81;
% if t>=0 & t<8
%  if t>=0 & t<1 
%     theta_d=pi/6*t^2 ;           theta_d_dot=pi/3*t ;      theta_d_dot_dot=pi/3;
%  elseif t>=1 & t<3
%     theta_d=-pi/6*(t-2)^2+pi/3 ; theta_d_dot=-pi/3*(t-2) ; theta_d_dot_dot=-pi/3;
%  elseif t>=3 & t<4
%     theta_d=pi/6*(t-4)^2 ;       theta_d_dot=pi/3*(t-4) ;  theta_d_dot_dot=pi/3;
%  elseif t>=4 & t<5
%     theta_d=-pi/6*(t-4)^2 ;      theta_d_dot=-pi/3*(t-4) ; theta_d_dot_dot=-pi/3;
%  elseif t>=5 & t<7
%     theta_d=pi/6*(t-6)^2-pi/3 ;  theta_d_dot=pi/3*(t-6) ;  theta_d_dot_dot=pi/3;
%  else 
%     theta_d=-pi/6*(t-8)^2 ;      theta_d_dot=-pi/3*(t-8);  theta_d_dot_dot=-pi/3;
%  end
%  r_desired=[0 0 0]'    ;              % reference's positions is not solved here
%  r_desired_dot=[0 0 0]'    ;          % reference's velocities is not solved here
%  r_desired_dot_dot=[1/200*g*tan(theta_d) -sqrt(3)/200*g*tan(theta_d) 0]'   ;       % reference's accelerations
%  r_desired_dot_dot_dot=[1/200*g*(1+tan(theta_d)^2)*theta_d_dot -sqrt(3)/200*g*(1+tan(theta_d)^2)*theta_d_dot 0]';      % jerk
%  r_desired_dot_dot_dot_dot=[1/200*g*(1+tan(theta_d)^2)*(2*tan(theta_d)*theta_d_dot^2+theta_d_dot_dot) -sqrt(3)/200*g*(1+tan(theta_d)^2)*(2*tan(theta_d)*theta_d_dot^2+theta_d_dot_dot) 0]' ; % snap
%  psi_desired=-pi/3 ;                      % reference's yaw angle
%  psi_desired_dot=0 ;                  % reference's change rate of yaw angle       
%  psi_desired_dot_dot=0;
%  
% elseif t>=8 & t<10 
% r_desired=[0 0 0]'    ;              % reference's positions 
% r_desired_dot=[0 0 0]'    ;          % reference's velocities
% r_desired_dot_dot=[0 0 0]'   ;       % reference's accelerations
% r_desired_dot_dot_dot=[0 0 0]';      % jerk
% r_desired_dot_dot_dot_dot=[0 0 0]' ; % snap
% if t>=8 & t<9
% psi_desired=-pi/3+pi/3*(t-8)^2 ;                      % reference's yaw angle
% psi_desired_dot=pi*2/3*(t-8);                  % reference's change rate of yaw angle       
% psi_desired_dot_dot=pi*2/3; 
% else
% psi_desired=-pi/3*(t-10)^2+pi/3 ;                      % reference's yaw angle
% psi_desired_dot=-pi*2/3*(t-10);                  % reference's change rate of yaw angle       
% psi_desired_dot_dot=-pi*2/3; 
% end
% 
% elseif t>=10 & t<18
%   if t>=10 & t<11 
%     theta_d=pi/6*(t-10)^2 ;           theta_d_dot=pi/3*(t-10) ;      theta_d_dot_dot=pi/3;
%  elseif t>=11 & t<13
%     theta_d=-pi/6*(t-12)^2+pi/3 ; theta_d_dot=-pi/3*(t-12) ; theta_d_dot_dot=-pi/3;
%  elseif t>=13 & t<14
%     theta_d=pi/6*(t-14)^2 ;       theta_d_dot=pi/3*(t-14) ;  theta_d_dot_dot=pi/3;
%  elseif t>=14 & t<15
%     theta_d=-pi/6*(t-14)^2 ;      theta_d_dot=-pi/3*(t-14) ; theta_d_dot_dot=-pi/3;
%  elseif t>=15 & t<17
%     theta_d=pi/6*(t-16)^2-pi/3 ;  theta_d_dot=pi/3*(t-16) ;  theta_d_dot_dot=pi/3;
%  else 
%     theta_d=-pi/6*(t-18)^2 ;      theta_d_dot=-pi/3*(t-18);  theta_d_dot_dot=-pi/3;
%  end
%  r_desired=[0 0 0]'    ;              % reference's positions is not solved here
%  r_desired_dot=[0 0 0]'    ;          % reference's velocities is not solved here
%  r_desired_dot_dot=[1/200*g*tan(theta_d) sqrt(3)/200*g*tan(theta_d) 0]'   ;       % reference's accelerations
%  r_desired_dot_dot_dot=[1/200*g*(1+tan(theta_d)^2)*theta_d_dot sqrt(3)/200*g*(1+tan(theta_d)^2)*theta_d_dot 0]';      % jerk
%  r_desired_dot_dot_dot_dot=[1/200*g*(1+tan(theta_d)^2)*(2*tan(theta_d)*theta_d_dot^2+theta_d_dot_dot) sqrt(3)/200*g*(1+tan(theta_d)^2)*(2*tan(theta_d)*theta_d_dot^2+theta_d_dot_dot) 0]' ; % snap
%  psi_desired=pi/3 ;                      % reference's yaw angle
%  psi_desired_dot=0 ;                  % reference's change rate of yaw angle       
%  psi_desired_dot_dot=0;  
%  
% elseif t>=18 & t<20
% r_desired=[0 0 0]'    ;              % reference's positions 
% r_desired_dot=[0 0 0]'    ;          % reference's velocities
% r_desired_dot_dot=[0 0 0]'   ;       % reference's accelerations
% r_desired_dot_dot_dot=[0 0 0]';      % jerk
% r_desired_dot_dot_dot_dot=[0 0 0]' ; % snap
% if t>=18 & t<19
% psi_desired=pi/3-pi/3*(t-18)^2 ;                      % reference's yaw angle
% psi_desired_dot=-pi*2/3*(t-18);                  % reference's change rate of yaw angle       
% psi_desired_dot_dot=-pi*2/3; 
% else
% psi_desired=pi/3*(t-20)^2-pi/3 ;                      % reference's yaw angle
% psi_desired_dot=pi*2/3*(t-20);                  % reference's change rate of yaw angle       
% psi_desired_dot_dot=pi*2/3; 
% end
% 
% elseif t>=20 & t<28
%  if t>=20 & t<21 
%     theta_d=pi/6*(t-20)^2 ;           theta_d_dot=pi/3*(t-20) ;      theta_d_dot_dot=pi/3;
%  elseif t>=21 & t<23
%     theta_d=-pi/6*(t-22)^2+pi/3 ; theta_d_dot=-pi/3*(t-22) ; theta_d_dot_dot=-pi/3;
%  elseif t>=23 & t<24
%     theta_d=pi/6*(t-24)^2 ;       theta_d_dot=pi/3*(t-24) ;  theta_d_dot_dot=pi/3;
%  elseif t>=24 & t<25
%     theta_d=-pi/6*(t-24)^2 ;      theta_d_dot=-pi/3*(t-24) ; theta_d_dot_dot=-pi/3;
%  elseif t>=25 & t<27
%     theta_d=pi/6*(t-26)^2-pi/3 ;  theta_d_dot=pi/3*(t-26) ;  theta_d_dot_dot=pi/3;
%  else 
%     theta_d=-pi/6*(t-28)^2 ;      theta_d_dot=-pi/3*(t-28);  theta_d_dot_dot=-pi/3;
%  end
%  r_desired=[0 0 0]'    ;              % reference's positions is not solved here
%  r_desired_dot=[0 0 0]'    ;          % reference's velocities is not solved here
%  r_desired_dot_dot=[1/200*g*tan(theta_d) -sqrt(3)/200*g*tan(theta_d) 0]'   ;       % reference's accelerations
%  r_desired_dot_dot_dot=[1/200*g*(1+tan(theta_d)^2)*theta_d_dot -sqrt(3)/200*g*(1+tan(theta_d)^2)*theta_d_dot 0]';      % jerk
%  r_desired_dot_dot_dot_dot=[1/200*g*(1+tan(theta_d)^2)*(2*tan(theta_d)*theta_d_dot^2+theta_d_dot_dot) -sqrt(3)/200*g*(1+tan(theta_d)^2)*(2*tan(theta_d)*theta_d_dot^2+theta_d_dot_dot) 0]' ; % snap
%  psi_desired=-pi/3 ;                      % reference's yaw angle
%  psi_desired_dot=0 ;                      % reference's change rate of yaw angle       
%  psi_desired_dot_dot=0; 
%  
% elseif t>=28 & t<30
% r_desired=[0 0 0]'    ;              % reference's positions 
% r_desired_dot=[0 0 0]'    ;          % reference's velocities
% r_desired_dot_dot=[0 0 0]'   ;       % reference's accelerations
% r_desired_dot_dot_dot=[0 0 0]';      % jerk
% r_desired_dot_dot_dot_dot=[0 0 0]' ; % snap
% if t>=28 & t<29
% psi_desired=-pi/3+pi/3*(t-28)^2 ;                      % reference's yaw angle
% psi_desired_dot=pi*2/3*(t-28);                  % reference's change rate of yaw angle       
% psi_desired_dot_dot=pi*2/3; 
% else
% psi_desired=-pi/3*(t-30)^2+pi/3 ;                      % reference's yaw angle
% psi_desired_dot=-pi*2/3*(t-30);                  % reference's change rate of yaw angle       
% psi_desired_dot_dot=-pi*2/3; 
% end
% 
% else
% if t>=30 & t<31 
%     theta_d=pi/6*(t-30)^2 ;           theta_d_dot=pi/3*(t-30) ;      theta_d_dot_dot=pi/3;
%  elseif t>=31 & t<33
%     theta_d=-pi/6*(t-32)^2+pi/3 ; theta_d_dot=-pi/3*(t-32) ; theta_d_dot_dot=-pi/3;
%  elseif t>=33 & t<34
%     theta_d=pi/6*(t-34)^2 ;       theta_d_dot=pi/3*(t-34) ;  theta_d_dot_dot=pi/3;
%  elseif t>=34 & t<35
%     theta_d=-pi/6*(t-34)^2 ;      theta_d_dot=-pi/3*(t-34) ; theta_d_dot_dot=-pi/3;
%  elseif t>=35 & t<37
%     theta_d=pi/6*(t-36)^2-pi/3 ;  theta_d_dot=pi/3*(t-36) ;  theta_d_dot_dot=pi/3;
%  else 
%     theta_d=-pi/6*(t-38)^2 ;      theta_d_dot=-pi/3*(t-38);  theta_d_dot_dot=-pi/3;
%  end
%  r_desired=[0 0 0]'    ;              % reference's positions is not solved here
%  r_desired_dot=[0 0 0]'    ;          % reference's velocities is not solved here
%  r_desired_dot_dot=[1/200*g*tan(theta_d) sqrt(3)/200*g*tan(theta_d) 0]'   ;       % reference's accelerations
%  r_desired_dot_dot_dot=[1/200*g*(1+tan(theta_d)^2)*theta_d_dot sqrt(3)/200*g*(1+tan(theta_d)^2)*theta_d_dot 0]';      % jerk
%  r_desired_dot_dot_dot_dot=[1/200*g*(1+tan(theta_d)^2)*(2*tan(theta_d)*theta_d_dot^2+theta_d_dot_dot) sqrt(3)/200*g*(1+tan(theta_d)^2)*(2*tan(theta_d)*theta_d_dot^2+theta_d_dot_dot) 0]' ; % snap
%  psi_desired=pi/3 ;                      % reference's yaw angle
%  psi_desired_dot=0 ;                  % reference's change rate of yaw angle       
%  psi_desired_dot_dot=0;  
%
% end
%% ------------xi hu da xue---------
% g=9.81;
% if t>=0 & t<8
%  if t>=0 & t<1 
%     theta_d=pi/6*t^2 ;           theta_d_dot=pi/3*t ;      theta_d_dot_dot=pi/3;
%  elseif t>=1 & t<3
%     theta_d=-pi/6*(t-2)^2+pi/3 ; theta_d_dot=-pi/3*(t-2) ; theta_d_dot_dot=-pi/3;
%  elseif t>=3 & t<4
%     theta_d=pi/6*(t-4)^2 ;       theta_d_dot=pi/3*(t-4) ;  theta_d_dot_dot=pi/3;
%  elseif t>=4 & t<5
%     theta_d=-pi/6*(t-4)^2 ;      theta_d_dot=-pi/3*(t-4) ; theta_d_dot_dot=-pi/3;
%  elseif t>=5 & t<7
%     theta_d=pi/6*(t-6)^2-pi/3 ;  theta_d_dot=pi/3*(t-6) ;  theta_d_dot_dot=pi/3;
%  else % t>=7 & t<8
%     theta_d=-pi/6*(t-8)^2 ;      theta_d_dot=-pi/3*(t-8);  theta_d_dot_dot=-pi/3;
%  end
%  r_desired=[0 0 0]'    ;              % reference's positions is not solved here
%  r_desired_dot=[0 0 0]'    ;          % reference's velocities is not solved here
%  r_desired_dot_dot=[1/100*g*tan(theta_d) 0 0]'   ;       % reference's accelerations
%  r_desired_dot_dot_dot=[1/100*g*(1+tan(theta_d)^2)*theta_d_dot 0 0]';      % jerk
%  r_desired_dot_dot_dot_dot=[1/100*g*(1+tan(theta_d)^2)*(2*tan(theta_d)*theta_d_dot^2+theta_d_dot_dot) 0 0]' ; % snap
%  psi_desired=0 ;                      % reference's yaw angle
%  psi_desired_dot=0 ;                  % reference's change rate of yaw angle       
%  psi_desired_dot_dot=0;
%  
% elseif t>=8 & t<10
% r_desired=[0 0 0]'    ;              % reference's positions is not solved here
% r_desired_dot=[0 0 0]'    ;          % reference's velocities is not solved here
% r_desired_dot_dot=[0 0 0]'   ;       % reference's accelerations
% r_desired_dot_dot_dot=[0 0 0]';      % jerk
% r_desired_dot_dot_dot_dot=[0 0 0]' ; % snap
% if t>=8 & t<9
% psi_desired=pi/4*(t-8)^2 ;                      % reference's yaw angle
% psi_desired_dot=pi/2*(t-8);                  % reference's change rate of yaw angle       
% psi_desired_dot_dot=pi/2; 
% else % t>=9 & t<10
% psi_desired=-pi/4*(t-10)^2+pi/2 ;                      % reference's yaw angle
% psi_desired_dot=-pi/2*(t-10);                  % reference's change rate of yaw angle       
% psi_desired_dot_dot=-pi/2; 
% end
% 
% elseif t>=10 & t<12
% if t>=10 & t<11
%  r_desired=[0 0 -1/4*(t-10)^2]'    ;              % reference's positions 
%  r_desired_dot=[0 0 -1/2*(t-8)]'    ;          % reference's velocities
%  r_desired_dot_dot=[0 0 -1/2]'   ;       % reference's accelerations
%  r_desired_dot_dot_dot=[0 0 0]';      % jerk
%  r_desired_dot_dot_dot_dot=[0 0 0]' ; % snap
% else % t>=11 & t<12
%  r_desired=[0 0 1/4*(t-12)^2+1/2]'    ;              % reference's positions 
%  r_desired_dot=[0 0 1/2*(t-12)]'    ;          % reference's velocities 
%  r_desired_dot_dot=[0 0 1/2]'   ;       % reference's accelerations
%  r_desired_dot_dot_dot=[0 0 0]';      % jerk
%  r_desired_dot_dot_dot_dot=[0 0 0]' ; % snap
% end
%  psi_desired=pi/2;                      % reference's yaw angle
%  psi_desired_dot=0 ;                  % reference's change rate of yaw angle       
%  psi_desired_dot_dot=0;
%  
% elseif t>=12 & t<20
% if t>=12 & t<13 
%     phi_d=-pi/6*(t-12)^2 ;           phi_d_dot=-pi/3*(t-12) ;      phi_d_dot_dot=-pi/3;
%  elseif t>=13 & t<15
%     phi_d=pi/6*(t-14)^2-pi/3 ;       phi_d_dot=pi/3*(t-14) ;       phi_d_dot_dot=pi/3;
%  elseif t>=15 & t<16
%     phi_d=-pi/6*(t-16)^2 ;           phi_d_dot=-pi/3*(t-16) ;      phi_d_dot_dot=-pi/3;
%  elseif t>=16 & t<17
%     phi_d=pi/6*(t-16)^2 ;            phi_d_dot=pi/3*(t-16) ;       phi_d_dot_dot=pi/3;
%  elseif t>=17 & t<19
%     phi_d=-pi/6*(t-18)^2+pi/3 ;      phi_d_dot=-pi/3*(t-18) ;      phi_d_dot_dot=-pi/3;
%  else % t>=19 & t<20
%     phi_d=pi/6*(t-20)^2 ;            phi_d_dot=pi/3*(t-20);        phi_d_dot_dot=pi/3;
% end
%  r_desired=[0 0 0]'    ;              % reference's positions is not solved here
%  r_desired_dot=[0 0 0]'    ;          % reference's velocities is not solved here
%  r_desired_dot_dot=[1/100*g*tan(phi_d) 0 0]'   ;       % reference's accelerations
%  r_desired_dot_dot_dot=[1/100*g*(1+tan(phi_d)^2)*phi_d_dot 0 0]';      % jerk
%  r_desired_dot_dot_dot_dot=[1/100*g*(1+tan(phi_d)^2)*(2*tan(phi_d)*phi_d_dot^2+phi_d_dot_dot) 0 0]' ; % snap
%  psi_desired=pi/2 ;                      % reference's yaw angle
%  psi_desired_dot=0 ;                  % reference's change rate of yaw angle       
%  psi_desired_dot_dot=0;
%  
% elseif t>=20 & t<22
% r_desired=[0 0 0]'    ;              % reference's positions is not solved here
% r_desired_dot=[0 0 0]'    ;          % reference's velocities is not solved here
% r_desired_dot_dot=[0 0 0]'   ;       % reference's accelerations
% r_desired_dot_dot_dot=[0 0 0]';      % jerk
% r_desired_dot_dot_dot_dot=[0 0 0]' ; % snap
% if t>=20 & t<21
% psi_desired=pi/2-pi/4*(t-20)^2 ;                      % reference's yaw angle
% psi_desired_dot=-pi/2*(t-20);                  % reference's change rate of yaw angle       
% psi_desired_dot_dot=-pi/2; 
% else % t>=21 & t<22
% psi_desired=pi/4*(t-22)^2 ;                      % reference's yaw angle
% psi_desired_dot=pi/2*(t-22);                  % reference's change rate of yaw angle       
% psi_desired_dot_dot=pi/2; 
% end
% 
% else
% if t>=22 & t<23
%  r_desired=[0 0 -1/2*(t-22)^2-1/2]'    ;              % reference's positions 
%  r_desired_dot=[0 0 -(t-22)]'    ;          % reference's velocities
%  r_desired_dot_dot=[0 0 -1]'   ;       % reference's accelerations
%  r_desired_dot_dot_dot=[0 0 0]';      % jerk
%  r_desired_dot_dot_dot_dot=[0 0 0]' ; % snap
% else % t>=23 & t<24
%  r_desired=[0 0 1/2*(t-24)^2-3/2]'    ;              % reference's positions 
%  r_desired_dot=[0 0 (t-24)]'    ;          % reference's velocities 
%  r_desired_dot_dot=[0 0 1]'   ;       % reference's accelerations
%  r_desired_dot_dot_dot=[0 0 0]';      % jerk
%  r_desired_dot_dot_dot_dot=[0 0 0]' ; % snap
% end
%  psi_desired=0 ;                      % reference's yaw angle
%  psi_desired_dot=0 ;                  % reference's change rate of yaw angle       
%  psi_desired_dot_dot=0;
% 
% end
